simulink model "HGO_gfr"  (R2017a)
settings: Solver=VariableStepAuto  StartTime=0.0  StopTime=5  RelTol=1e-3
values from neighbouring files (symbols this model uses):
  Ar_mod = [zeros(n) eye(n); zeros(n) zeros(n)]    [HGO_grf_init.m]
  beta = 0    [Init_4DOF_grf_HGO_ctpid_sf.m]
  BodyContactPositions = [ contact_point_h, contact_point_t ]    [Init_4DOF_grf_HGO_ctpid_sf.m]
  Br_mod = [zeros(n); eye(n)]    [HGO_grf_init.m]
  Cr_mod = [eye(n) zeros(n); zeros(n) eye(n)]    [HGO_grf_init.m]
  grf_init = 0    [HGO_grf_init.m]
  h = [ ez -ey -ey -ey ]    [Init_4DOF_grf_HGO_ctpid_sf.m]
  Hmu_mod = [eye(n)/Mu_mod zeros(n); zeros(n) eye(n)/Mu_mod^2 ]    [HGO_grf_init.m]
  joint_type = [ 1 0 0 0 ]    [Init_4DOF_grf_HGO_ctpid_sf.m]
  k_b = 50000    [Init_4DOF_grf_HGO_ctpid_sf.m]
  L = [ l_base_hip l_hip_thigh l_thigh_shin l_shin_foot ]    [Init_4DOF_grf_HGO_ctpid_sf.m]
  L_hgo_mod = [5*eye(n);10*eye(n)]    [HGO_grf_init.m]
  s_z = 1    [Init_4DOF_grf_HGO_ctpid_sf.m]
settings Model: Creator=igricart  LastModifiedBy=igricart

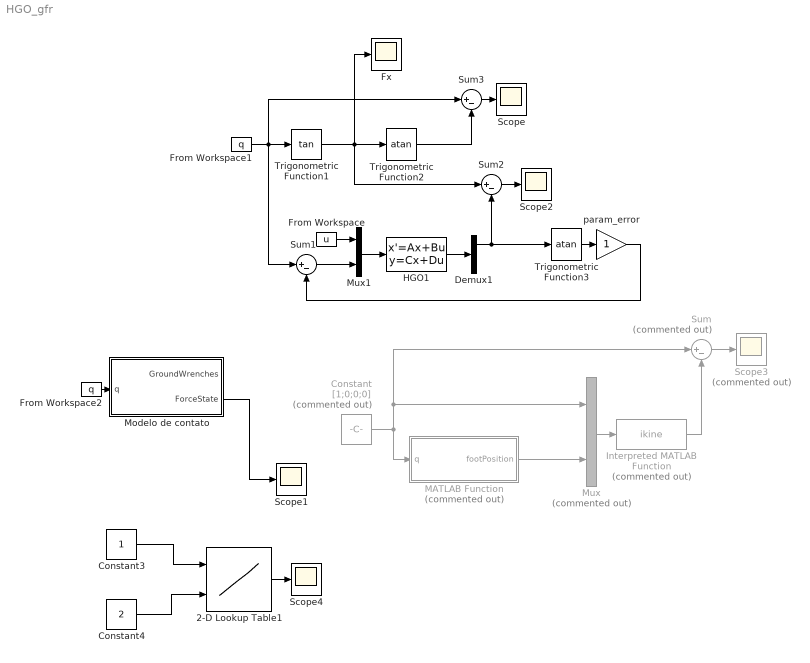
== system HGO_gfr ==
  2-D Lookup Table1 : Lookup_n-D  BreakpointsForDimension1=[1:3]  BreakpointsForDimension2=[1:3]  Table=[ 1 2 3; 4 5 6; 7 8 9]  InternalRulePriority=Speed  RndMeth=Simplest  InputSameDT=on
  Constant : Constant  Commented=on  Value=[1;0;0;0]
  Constant3 : Constant
  Constant4 : Constant  Value=2
  Demux1 : Demux  Outputs=2
  From Workspace : FromWorkspace  VariableName=u  SampleTime=0
  From Workspace1 : FromWorkspace  VariableName=q  SampleTime=0
  From Workspace2 : FromWorkspace  VariableName=q  SampleTime=0
  Fx : Scope
  HGO1 : StateSpace  A=Ar_mod  B=[Br_mod Hmu_mod*L_hgo_mod]  C=Cr_mod  D=zeros(8,8)  X0=grf_init
  Interpreted MATLAB Function : MATLABFcn  Commented=on  MATLABFcn=ikine
  MATLAB Function : MATLAB Function  Commented=on  TreatAsAtomicUnit=on
  Modelo de contato : MATLAB Function  TreatAsAtomicUnit=on
  Mux : Mux  Commented=on  Inputs=2
  Mux1 : Mux  Inputs=2
  Scope{,1..2,4} (4 alike) : Scope
  Scope3 : Scope  Commented=on
  Sum : Sum  Commented=on  Inputs=|+-
  Sum1 : Sum  Inputs=|+-
  Sum2 : Sum  Inputs=|+-
  Sum3 : Sum  Inputs=|+-
  Trigonometric Function1 : Trigonometry  Operator=tan
  Trigonometric Function2 : Trigonometry  Operator=atan
  Trigonometric Function3 : Trigonometry  Operator=atan
  param_error : Gain
  wires:
  Sum3/1 -> Scope/1
  Trigonometric Function1/1 -> Fx/1, Sum2/1, Trigonometric Function2/1
  From Workspace/1 -> Mux1/1
  Demux1/1 -> Sum2/2, Trigonometric Function3/1
  From Workspace1/1 -> Sum3/1, Sum1/1, Trigonometric Function1/1
  Mux1/1 -> HGO1/1
  Sum2/1 -> Scope2/1
  Trigonometric Function2/1 -> Sum3/2
  Sum1/1 -> Mux1/2
  HGO1/1 -> Demux1/1
  param_error/1 -> Sum1/2
  Trigonometric Function3/1 -> param_error/1
  From Workspace2/1 -> Modelo de contato/1(q)
  Modelo de contato/2(ForceState) -> Scope1/1
  Constant/1 -> Mux/1, Sum/1, MATLAB Function/1(q)
  MATLAB Function/1(footPosition) -> Mux/2
  Interpreted MATLAB Function/1 -> Sum/2
  Sum/1 -> Scope3/1
  Mux/1 -> Interpreted MATLAB Function/1
  Constant3/1 -> 2-D Lookup Table1/1
  Constant4/1 -> 2-D Lookup Table1/2
  2-D Lookup Table1/1 -> Scope4/1

== matlab function HGO_gfr/Modelo de contato ==
  data: GroundWrenches output; q input; BodyContactPositions parameter; s_z parameter; L parameter; h parameter; beta parameter; k_b parameter; joint_type parameter; ForceState output
function [ GroundWrenches, ForceState ] = fcn( q, BodyContactPositions, s_z, L, h, beta,  k_b, joint_type )
% function BodyContactWrenches = fcn( t, q, L, h, BodyContactPositions, joint_type, sz, beta, kb)
% Esta função calcula as forças de contato com o chão

[ GroundWrenches, ForceState ] = ground_model( q, BodyContactPositions, s_z, L, h, beta,  k_b, joint_type );

== matlab function HGO_gfr/MATLAB Function ==
  data: q input; footPosition output; L parameter; BodyContactPositions parameter
function footPosition = fcn( q, L, BodyContactPositions)

%% Leg parameters according to Fakoorian paper
contact_point_h = BodyContactPositions(:,1);
contact_point_t = BodyContactPositions(:,2);

l2 = L(3,3);
l3 = L(3,4);
ah = contact_point_h(3);
aH = norm(contact_point_h);
aT = norm(contact_point_t);

%% Equations

anal_z_h = q(1) + l2 * cos( q(2) ) + l3 * ( cos( q(2) + q(3) ) ) ...
+ aH * cos( q(2) + q(3) + q(4) + ( - acos( ah / aH ) ) );

anal_z_t = q(1) + l2 * cos( q(2) ) + l3 * ( cos( q(2) + q(3) ) ) ...
+ aT * cos( q(2) + q(3) + q(4) + ( acos( ah / aT ) ) );

footPosition = [anal_z_h ;anal_z_t ];
end
